simulink model "force_motor_control"  (R2024b)
settings: Solver=VariableStepAuto  StartTime=0.0  StopTime=10.0  RelTol=1e-3
values from neighbouring files (symbols this model uses):
  b = 2 * zeta_min * sqrt(k_max * m_v)    [direct-parameter-solve.m]    (also in direct_parameter_solve.m; force_motor_control_script.m = 150; untitled.m = 5)
  k = 200e3    (= 200000)    [force_motor_control_script.m]    (also in untitled.m = 100)
  m_v = k_max / omega_n^2    (= 1378.125)    [direct-parameter-solve.m]    (also in direct_parameter_solve.m; force_motor_control_script.m = 2; untitled.m = 1)
settings Model: Creator=et  LastModifiedBy=et

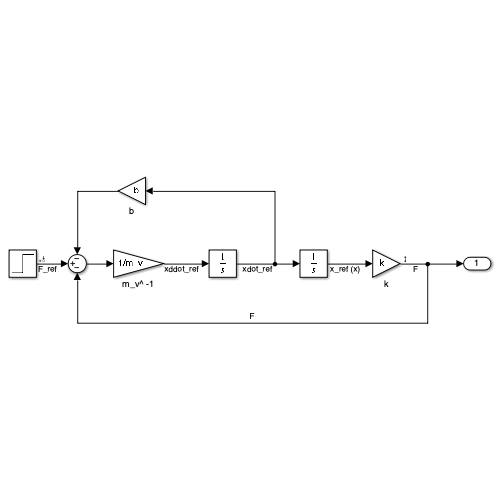
[thumbnail: Simulink's stored preview of the top-level diagram]
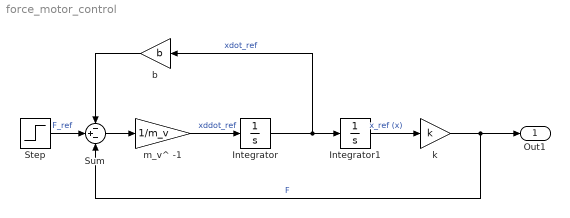
== system force_motor_control ==
  Integrator : Integrator
  Integrator1 : Integrator
  Step : Step  After=2000  SampleTime=0
  Sum : Sum  Inputs=-+-
  b : Gain  Gain=b
  k : Gain  Gain=k
  m_v^ -1 : Gain  Gain=1/m_v
  Out1 : Outport
  wires:
  Sum/1 -> m_v^ -1/1
  Step/1 -> Sum/2  "F_ref"
  m_v^ -1/1 -> Integrator/1  "xddot_ref"
  Integrator/1 -> Integrator1/1, b/1  "xdot_ref"
  b/1 -> Sum/1
  Integrator1/1 -> k/1  "x_ref (x)"
  k/1 -> Sum/3, Out1/1  "F"
